simulink model "HybridControllerD3D3_1Act"  (Simulink 8.1)
settings: Solver=FixedStepDiscrete  SolverMode=SingleTasking  StartTime=0.0  StopTime=inf  FixedStep=0.001  MaxStep=.1  RelTol=1e-3
PreLoadFcn:
  | initializeSimulation
PostLoadFcn:
  | , if any(exist('dsrtsu_mdlpostloadfcn', 'file') == [2, 3, 6]), try dsrtsu_mdlpostloadfcn('Execute', bdroot); catch fprintf('Error in PostLoadFcn (dsrtsu_mdlpostloadfcn) for model "%s":\n %s\n', bdroot, lasterr); end, end,
values from neighbouring files (symbols this model uses):
  nAct = 1    [initializeSimulation.m]
  newTarget = 0    [initializeSimulation.m]
  targDsp = zeros(1,nAct)    [initializeSimulation.m]
undefined symbols (not defined in the file): HybridCtrlParameters
libraries: simulink x4, HybridSimLib x3, rtilib1104 x2
CloseFcn:
  | rtwprivate ssgencode ModelCloseRequest HybridController2
settings Model: DSRTSU_INTERNAL_RTI_VER=420  DSRTSU_INTERNAL_RTI_TYPE=rti1104  DSRTSU_INTERNAL_RTIFPGA=10  Creator=Andreas Schellenberg  LastModifiedBy=RTHS Experimentalist  ExtModeAutoUpdateStatusClock=off  TunableVars=newTarget,targDsp  TunableVarsStorageClass=ExportedGlobal,ExportedGlobal  TunableVarsTypeQualifier=volatile,volatile  BufferReuse=off
settings DataIOCC: LimitDataPoints=off  SaveOutput=off  SignalLogging=off  SaveTime=off  SignalLoggingName=sigsOut
settings OptimizationCC: BlockReduction=off  ConditionallyExecuteInputs=off  InlineParams=on  OptimizeBlockIOStorage=off  BufferReuse=off  ExpressionFolding=off  FoldNonRolledExpr=off  LocalBlockOutputs=off  StateBitsets=on  DataBitsets=on  UseTempVars=on  InitFltsAndDblsToZero=on  EfficientFloat2IntCast=on
settings DebuggingCC: SaveWithParameterizedLinksMsg=none  CheckSSInitialOutputMsg=off  SolverPrmCheckMsg=none  StrictBusMsg=None
settings HardwareCC: ProdIntDivRoundTo=Zero  ProdEndianess=BigEndian  ProdHWDeviceType=Generic->Custom  TargetIntDivRoundTo=Zero  TargetEndianess=BigEndian  TargetHWDeviceType=Generic->Custom
settings SFSimCC: SimCustomHeaderCode="#include \"PredictorCorrector.h\""  SimUserSources=PredictorCorrector.c  SimParseCustomCode=off  SimBuildMode=sf_nonincremental_build
settings RTWCC: SystemTargetFile=rti1104.tlc  MakeCommand=make_rti  TemplateMakefile=rti1104.tmf  Description=dSPACE DS1104 Hardware Platform  ProcessScript=rti1104_make_rtw_hook  CustomHeaderCode="#include \"PredictorCorrector.h\""  CustomSource=PredictorCorrector.c  IncludeERTFirstTime=on
settings STFCustomTargetCC: TargetFcnLib=ansi_tfl_tmw.mat  CodeReplacementLibrary=ANSI_C  ParMdlRefBuildCompliant=on  GeneratePreprocessorConditionals=Disable all  LogVarNameModifier=none  SystemTargetFile=rti1104.tlc
settings GRTTargetCC: TargetFcnLib=ansi_tfl_tmw.mat  CompOptLevelCompliant=off  ConcurrentExecutionCompliant=off  LogVarNameModifier=none  MatFileLogging=off  ExtModeMexFile=noextcomm
settings CustomProperty: DataType=RTWOptions_EnumType_C__Program Files_dSPACE RCPHIL 2013-A_MATLAB_RTI_RTI1104_TLC_rti1104_1InitialSimState  Value=STOP
settings EnumStrPairs: String=RUN

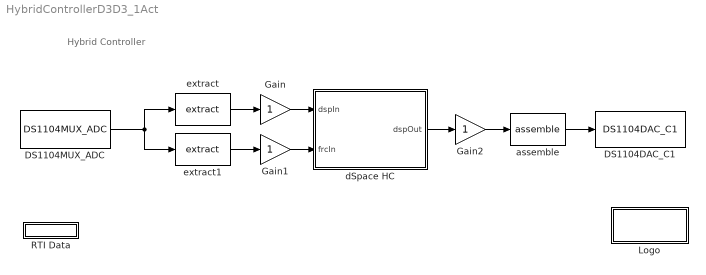
== system HybridControllerD3D3_1Act ==
  note: Hybrid Controller
  DS1104DAC_C1 : rtilib1104/DS1104 MASTER PPC/DS1104DAC_C1  ChannelNo=1  InitValue=0  TermMode=0  TermValue=0  Reserved1=[]  Reserved2=[]  Reserved3=[]  Reserved4=[]  DialogFcn=gui1104dac  UnitName={ 'DS1104DAC_C'}  UnitValues={ 1 }  DSProperties=struct('RTI',struct('Version',uint32(1),'BlockType',struct('isSLSource',uint8(0),'isSLSink',uint8(1),'isHWSource',uint8(0),'isHWSink',uint8(1),'isSetup',uint8(0),'isInline',uint8(1),'isNonInline',uint8(0),'isInterrupt',uint8(0),'isChannelwise',uint8(1)),'IOBoardType','DS1104MASTER','UnitType','DAC','Identifier','DAC','DialogType','ML','BlockSet','NONE','SlaveProcessor','NONE'))
  DS1104MUX_ADC : rtilib1104/DS1104 MASTER PPC/DS1104MUX_ADC  ChannelNos=[1 3]  TriggerMode=0  Reserved1=[]  Reserved2=[]  Reserved3=[]  Reserved4=[]  DialogFcn=gui1104mux_adc  UnitName={ 'DS1104MUX_ADC' }  UnitValues={ [] }  DSProperties=struct('RTI',struct('Version',uint32(1),'BlockType',struct('isSLSource',uint8(1),'isSLSink',uint8(0),'isHWSource',uint8(1),'isHWSink',uint8(0),'isSetup',uint8(0),'isInline',uint8(1),'isNonInline',uint8(0),'isInterrupt',uint8(0),'isChannelwise',uint8(0)),'IOBoardType','DS1104MASTER','UnitType','ADC','Identifier','ADCMUX','DialogType','ML','BlockSet','NONE','SlaveProcessor','NONE'))
  Gain : Gain  SaturateOnIntegerOverflow=on  OutDataTypeStr=Inherit: Same as input  ParamDataTypeStr=Inherit: Same as input
  Gain1 : Gain  SaturateOnIntegerOverflow=on  OutDataTypeStr=Inherit: Same as input  ParamDataTypeStr=Inherit: Same as input
  Gain2 : Gain  SaturateOnIntegerOverflow=on  OutDataTypeStr=Inherit: Same as input  ParamDataTypeStr=Inherit: Same as input
  Logo : Subsystem  mask(dSPACE){EmptyParameter=[]}
      mask prompts: EmptyParameter "Mask Parameter 1:"
      settings: OpenFcn=;
      mask Display: image(imread('rti_mdl_dslogo.tif'));
  RTI Data : Subsystem  Tag=struct('RTIDataServer',struct('RTIDataServerVs','2','RTIModelDescription','struct(''main'',''HybridControllerD3D3_1Act'',''sub'','''',''isMp'',0)'))  LoadFcn="if exist('rtidc'), try,  rtidc('DataHostBlockClbLoad', gcbh); catch, disp(['Warning: ''LoadFcn'' for RTI Data block failed: ' lasterr]); end, end,"  mask(RTI_DATA_HOST){}
      mask help:
      | RTI Data Block.
      | This block is used by RTI to store internal model-dependent data.
      | Please keep this block on the root level of the model. Deleting this block will result in data loss.
      |
      | NEVER DELETE OR COPY THIS BLOCK!
      settings: CopyFcn="if exist('rtidc'), try,  rtidc('DataHostBlockClbCopy', gcbh); catch, disp(['Warning: ''CopyFcn'' for RTI Data block failed: ' lasterr]); end, end,"  DeleteFcn="if exist('rtidc'), try,  rtidc('DataHostBlockClbDelete', gcbh); catch, disp(['Warning: ''DeleteFcn'' for RTI Data block failed: ' lasterr]); end, end,"  ModelCloseFcn="if exist('rtidc'), try,  rtidc('DataHostBlockClbModelClose', gcbh); catch, disp(['Warning: ''ModelCloseFcn'' for RTI Data block failed: ' lasterr]); end, end,"  PreSaveFcn="if exist('rtidc'), try,  rtidc('DataHostBlockClbPreSave', gcbh); catch, disp(['Warning: ''PreSaveFcn'' for RTI Data block failed: ' lasterr]); end, end,"  PostSaveFcn="if exist('rtidc'), try,  rtidc('DataHostBlockClbPostSave', gcbh); catch, disp(['Warning: ''PostSaveFcn'' for RTI Data block failed: ' lasterr]); end, end,"  NameChangeFcn="if exist('rtidc'), try,  rtidc('DataHostBlockClbNameChange', gcbh); catch, disp(['Warning: ''NameChangeFcn'' for RTI Data block failed: ' lasterr]); end, end,"
      mask Help:
      | RTI Data Block.
      | This block is used by RTI to store internal model-dependent data.
      | Please keep this block on the root level of the model. Deleting this block will result in data loss.
      | 
      | NEVER DELETE OR COPY THIS BLOCK!
      mask Display:
      | text(0.5, 0.5, 'RTI Data', 'HorizontalAlignment', 'center');
      | plot([1 0]);
  assemble : HybridSimLib/Signal Routing/assemble  id=1  size=nAct
  dSpace HC : Subsystem  mask(Hybrid Controller: D3/D3){nAct=1, dtInt=HybridCtrlParameters.dtInt, dtSim=HybridCtrlParameters.dtSim, dtCon=HybridCtrlParameters.dtCon, N=HybridCtrlParameters.N, iDelay=HybridCtrlParameters.iDelay, dspLim=HybridCtrlParameters.dspLim, velLim=HybridCtrlParameters.velLim}
      mask prompts: nAct "Number of Actuators: nAct"; dtInt "Integration time step: dtInt"; dtSim "Simulation time step: dtSim"; dtCon "Controller time step: dtCon"; N "Maximum number of substeps: N"; iDelay "Number of delay steps: iDelay"; dspLim "Displacement limit: dspLim"; velLim "Velocity limit: velLim"
      mask help: Hybrid Controller using C0-continuous cubic Lagrange interpolation for prediction and correction
      mask Display: disp('dSpace\nHybrid Controller\n(D3/D3)')
  extract : HybridSimLib/Signal Routing/extract  id=1  size=2*nAct
  extract1 : HybridSimLib/Signal Routing/extract  id=2  size=2*nAct
  wires:
  dSpace HC/1(dspOut) -> Gain2/1
  Gain/1 -> dSpace HC/1(dspIn)
  Gain1/1 -> dSpace HC/2(frcIn)
  DS1104MUX_ADC/1 -> extract/1, extract1/1
  Gain2/1 -> assemble/1
  extract/1 -> Gain/1
  extract1/1 -> Gain1/1
  assemble/1 -> DS1104DAC_C1/1

== system HybridControllerD3D3_1Act/Logo ==
  note: $Workfile: demo1104_analog.mdl $
  note: $Date: 2011-05-22 14:17:07 -0700 (Sun, 22 May 2011) $
  note: $Revision: 314 $

== system HybridControllerD3D3_1Act/RTI Data ==
  RTI Data Store : Subsystem  Tag="struct('private',struct('version',struct('dsVer',uint32(2),'dsVerCreation',uint32(2),'RTI',struct('ver','4.1a3','type','RTI1104')),'access',struct('type','Model','isPerm',1,'created',['13-Feb-2001 14:58:17'],'modified',['01-Oct-2013 23:15:47'],'location','')),'public',struct('main',struct('data',[]),'sub',struct('name',{{'HybridControllerD3D3_1Act'}},'data',{{struct('TH',struct('thTaskInfo',struct('taskType',{'TIMER','HWINT','TMRINT','SWINT','GLINT'},'tasksNumOf',{1,0,0,0,0},'srcIds',{{'TIMERA'},{},{},{},{}},'taskNames',{{['Timer Task 1']},{},{},{},{}})),'th_tc',struct('dataType','TASK','taskGroupId','','taskGroupList',{{}},'taskSchedulingPolicy','FCFS','taskType','TIMER','blkh',-1,'srcId','TIMERA','srcSgnName',['Timer A interrupt'],'srcCpuName','','taskName',['Timer Task 1  [0.001] s'],'taskNameDisplayExt','','smplTime',0.001,'smplTimeOffs',0,'hasFixedPriority',0,'priority',1,'hasFixedOvc',0,'ovcType',1,'ovcMax',0),'tc_th',struct('dataType','TASK','taskGroupId','','taskGroupList',{{}},'taskSchedulingPolicy','FCFS','taskType','TIMER','blkh',-1,'srcId','TIMERA','srcSgnName',['Timer A interrupt'],'srcCpuName','','taskName',['Timer Task 1  [0.001] s'],'taskNameDisplayExt','','smplTime',0.001,'smplTimeOffs',0,'hasFixedPriority',0,'priority',1,'hasFixedOvc',0,'ovcType',1,'ovcMax',0))}})))"  mask(RTI_DATA_STORE){}
      mask help:
      | RTI Data Store Block. This block is used by RTI to store internal model dependent data. Deleting this block will result in data loss.
      |
      | NEVER DELETE, COPY, OR MODIFY THIS BLOCK!
      mask Help:
      | RTI Data Store Block. This block is used by RTI to store internal model dependent data. Deleting this block will result in data loss.
      | 
      | NEVER DELETE, COPY, OR MODIFY THIS BLOCK!
      mask Display: text(0.5, 0.5, ' ', 'HorizontalAlignment', 'center');

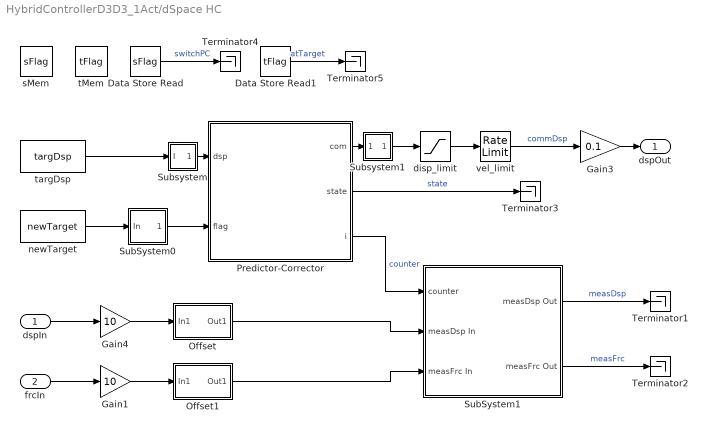
== system HybridControllerD3D3_1Act/dSpace HC ==
  dspIn : Inport
  frcIn : Inport  Port=2
  Data Store Read : DataStoreRead  DataStoreName=sFlag  SampleTime=dtCon
  Data Store Read1 : DataStoreRead  DataStoreName=tFlag  SampleTime=dtCon
  Gain1 : Gain  Gain=10  SaturateOnIntegerOverflow=on  OutDataTypeStr=Inherit: Same as input  ParamDataTypeStr=Inherit: Same as input
  Gain3 : Gain  Gain=0.1  SaturateOnIntegerOverflow=on  OutDataTypeStr=Inherit: Same as input  ParamDataTypeStr=Inherit: Same as input
  Gain4 : Gain  Gain=10  SaturateOnIntegerOverflow=on  OutDataTypeStr=Inherit: Same as input  ParamDataTypeStr=Inherit: Same as input
  Offset : Subsystem  mask(Signal Offset){nS=nAct, nOffset=1024, dt=dtCon}
      mask prompts: nS "Number of Signals: nS"; nOffset "Number of samples to initialize offset: nOffset"; dt "Sample time: dt"
      mask help: Offset signal by average of signal over initial number of samples
      mask Display: fprintf('Signal\nOffset')
  Offset1 : Subsystem  mask(Signal Offset){nS=nAct, nOffset=1024, dt=dtCon}
      mask prompts: nS "Number of Signals: nS"; nOffset "Number of samples to initialize offset: nOffset"; dt "Sample time: dt"
      mask help: Offset signal by average of signal over initial number of samples
      mask Display: fprintf('Signal\nOffset')
  Predictor-Corrector : Stateflow chart  TreatAsAtomicUnit=on
  SubSystem0 : Subsystem
  SubSystem1 : Subsystem
  Subsystem : Subsystem
      mask Display: disp('I/O')
  Subsystem1 : Subsystem
      mask Display: disp('I/O')
  Terminator{1..5} (5 alike) : Terminator
  disp_limit : Saturate  UpperLimit=dspLim  LowerLimit=-dspLim
  newTarget : Constant  Value=newTarget  OutDataTypeStr=uint32  SampleTime=dtCon
  sMem : DataStoreMemory  DataStoreName=sFlag  OutDataTypeStr=uint32
  tMem : DataStoreMemory  DataStoreName=tFlag  OutDataTypeStr=uint32
  targDsp : Constant  Value=targDsp  SampleTime=dtCon
  vel_limit : RateLimiter  RisingSlewLimit=velLim  FallingSlewLimit=-velLim
  dspOut : Outport
  wires:
  frcIn/1 -> Gain1/1
  dspIn/1 -> Gain4/1
  SubSystem1/2(measFrc Out) -> Terminator2/1  "measFrc"
  SubSystem1/1(measDsp Out) -> Terminator1/1  "measDsp"
  Predictor-Corrector/3(i) -> SubSystem1/1(counter)  "counter"
  Predictor-Corrector/2(state) -> Terminator3/1  "state"
  Offset/1(Out1) -> SubSystem1/2(measDsp In)
  newTarget/1 -> SubSystem0/1(In)
  targDsp/1 -> Subsystem/1(I)
  Offset1/1(Out1) -> SubSystem1/3(measFrc In)
  disp_limit/1 -> vel_limit/1
  vel_limit/1 -> Gain3/1  "commDsp"
  Predictor-Corrector/1(com) -> Subsystem1/1(In)
  Gain3/1 -> dspOut/1
  Gain4/1 -> Offset/1(In1)
  Gain1/1 -> Offset1/1(In1)
  Data Store Read/1 -> Terminator4/1  "switchPC"
  Data Store Read1/1 -> Terminator5/1  "atTarget"
  Subsystem1/1(Out) -> disp_limit/1
  SubSystem0/1(Out) -> Predictor-Corrector/2(flag)
  Subsystem/1(O) -> Predictor-Corrector/1(dsp)

== system HybridControllerD3D3_1Act/RTI Data/RTI Data Store ==
  RTI Data Store : Subsystem  mask(RTI_DATA_STORE){}
      mask help:
      | RTI Data Store Block. This block is used by RTI to store internal model dependent data. Deleting this block will result in data loss.
      |
      | NEVER DELETE, COPY, OR MODIFY THIS BLOCK!
      mask Help:
      | RTI Data Store Block. This block is used by RTI to store internal model dependent data. Deleting this block will result in data loss.
      | 
      | NEVER DELETE, COPY, OR MODIFY THIS BLOCK!
      mask Display: text(0.5, 0.5, ' ', 'HorizontalAlignment', 'center');

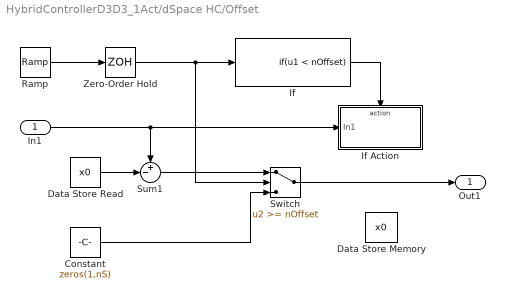
== system HybridControllerD3D3_1Act/dSpace HC/Offset ==
  In1 : Inport
  Constant : Constant  Value=zeros(1,nS)
  Data Store Memory : DataStoreMemory  DataStoreName=x0  InitialValue=zeros(1,nS)  OutDataTypeStr=double
  Data Store Read : DataStoreRead  DataStoreName=x0  SampleTime=dt
  If : If  IfExpression=u1 < nOffset  ShowElse=off
  If Action : Subsystem  TreatAsAtomicUnit=on
  Ramp : simulink/Sources/Ramp  slope=1/dt  start=0  X0=0
  Sum1 : Sum  Inputs=+-|  SaturateOnIntegerOverflow=on  InputSameDT=on  OutDataTypeStr=Inherit: Same as first input
  Switch : Switch  Threshold=nOffset  SaturateOnIntegerOverflow=on  InputSameDT=on
  Zero-Order Hold : ZeroOrderHold  SampleTime=dt
  Out1 : Outport
  wires:
  Switch/1 -> Out1/1
  Sum1/1 -> Switch/1
  Data Store Read/1 -> Sum1/2
  In1/1 -> If Action/1(In1), Sum1/1
  Constant/1 -> Switch/3
  Zero-Order Hold/1 -> Switch/2, If/1
  If/1 -> If Action/Action
  Ramp/1 -> Zero-Order Hold/1

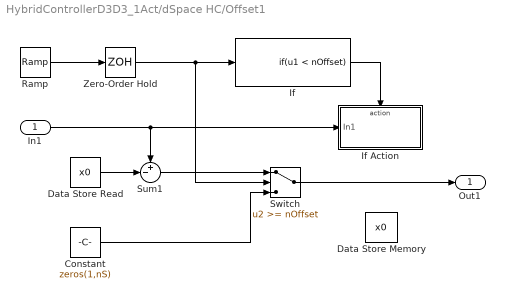
== system HybridControllerD3D3_1Act/dSpace HC/Offset1 ==
  In1 : Inport
  Constant : Constant  Value=zeros(1,nS)
  Data Store Memory : DataStoreMemory  DataStoreName=x0  InitialValue=zeros(1,nS)  OutDataTypeStr=double
  Data Store Read : DataStoreRead  DataStoreName=x0  SampleTime=dt
  If : If  IfExpression=u1 < nOffset  ShowElse=off
  If Action : Subsystem  TreatAsAtomicUnit=on
  Ramp : simulink/Sources/Ramp  slope=1/dt  start=0  X0=0
  Sum1 : Sum  Inputs=+-|  SaturateOnIntegerOverflow=on  InputSameDT=on  OutDataTypeStr=Inherit: Same as first input
  Switch : Switch  Threshold=nOffset  SaturateOnIntegerOverflow=on  InputSameDT=on
  Zero-Order Hold : ZeroOrderHold  SampleTime=dt
  Out1 : Outport
  wires:
  Switch/1 -> Out1/1
  Sum1/1 -> Switch/1
  Data Store Read/1 -> Sum1/2
  In1/1 -> If Action/1(In1), Sum1/1
  Constant/1 -> Switch/3
  Zero-Order Hold/1 -> Switch/2, If/1
  If/1 -> If Action/Action
  Ramp/1 -> Zero-Order Hold/1

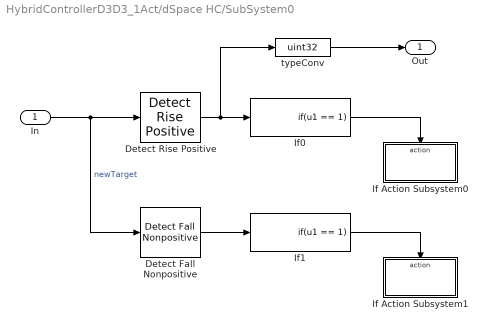
== system HybridControllerD3D3_1Act/dSpace HC/SubSystem0 ==
  In : Inport
  Detect Fall Nonpositive : simulink/Logic and Bit Operations/Detect Fall Nonpositive  vinit=0  InputProcessing=Inherited  OutDataTypeStr=uint8
  Detect Rise Positive : simulink/Logic and Bit Operations/Detect Rise Positive  vinit=0  InputProcessing=Inherited  OutDataTypeStr=uint8
  If Action Subsystem0 : Subsystem  TreatAsAtomicUnit=on
  If Action Subsystem1 : Subsystem  TreatAsAtomicUnit=on
  If0 : If  IfExpression=u1 == 1  ShowElse=off
  If1 : If  IfExpression=u1 == 1  ShowElse=off
  typeConv : DataTypeConversion  OutDataTypeStr=uint32  SaturateOnIntegerOverflow=on  RndMeth=Zero
  Out : Outport
  wires:
  In/1 -> Detect Rise Positive/1, Detect Fall Nonpositive/1  "newTarget"
  Detect Rise Positive/1 -> If0/1, typeConv/1
  Detect Fall Nonpositive/1 -> If1/1
  If1/1 -> If Action Subsystem1/Action
  If0/1 -> If Action Subsystem0/Action
  typeConv/1 -> Out/1

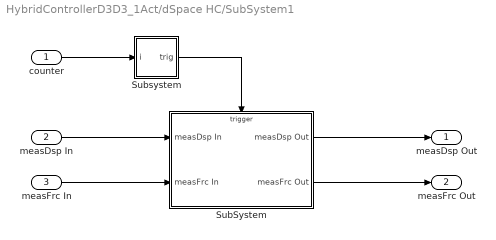
== system HybridControllerD3D3_1Act/dSpace HC/SubSystem1 ==
  counter : Inport
  measDsp In : Inport  Port=2
  measFrc In : Inport  Port=3
  SubSystem : Subsystem  TreatAsAtomicUnit=on
  Subsystem : Subsystem
  measDsp Out : Outport
  measFrc Out : Outport  Port=2
  wires:
  SubSystem/2(measFrc Out) -> measFrc Out/1
  measFrc In/1 -> SubSystem/2(measFrc In)
  SubSystem/1(measDsp Out) -> measDsp Out/1
  measDsp In/1 -> SubSystem/1(measDsp In)
  counter/1 -> Subsystem/1(i)
  Subsystem/1(trig) -> SubSystem/Trigger

== system HybridControllerD3D3_1Act/dSpace HC/Subsystem ==
  I : Inport  PortDimensions=nAct
  Dummy Aug : Mux  Inputs=[nAct 1]
  Dummy Zero : Constant  Value=0  OutDataTypeStr=double  SampleTime=dtCon
  O : Outport  PortDimensions=nAct+1
  wires:
  Dummy Zero/1 -> Dummy Aug/2
  I/1 -> Dummy Aug/1
  Dummy Aug/1 -> O/1

== system HybridControllerD3D3_1Act/dSpace HC/Subsystem1 ==
  In : Inport  PortDimensions=nAct+1
  Dummy Trn : Demux  Outputs=[nAct 1]
  Terminator3 : Terminator
  Out : Outport  PortDimensions=nAct
  wires:
  Dummy Trn/2 -> Terminator3/1
  Dummy Trn/1 -> Out/1
  In/1 -> Dummy Trn/1

== system HybridControllerD3D3_1Act/RTI Data/RTI Data Store/RTI Data Store ==
  RTI Data Store : Subsystem  mask(RTI_DATA_STORE){}
      mask help:
      | RTI Data Store Block. This block is used by RTI to store internal model dependent data. Deleting this block will result in data loss.
      |
      | NEVER DELETE, COPY, OR MODIFY THIS BLOCK!
      mask Help:
      | RTI Data Store Block. This block is used by RTI to store internal model dependent data. Deleting this block will result in data loss.
      | 
      | NEVER DELETE, COPY, OR MODIFY THIS BLOCK!
      mask Display: text(0.5, 0.5, ' ', 'HorizontalAlignment', 'center');

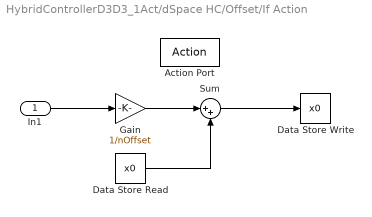
== system HybridControllerD3D3_1Act/dSpace HC/Offset/If Action ==
  In1 : Inport
  Action Port : ActionPort  PropagateVarSize=During execution  ActionType=then
  Data Store Read : DataStoreRead  DataStoreName=x0  SampleTime=dt
  Data Store Write : DataStoreWrite  DataStoreName=x0
  Gain : Gain  Gain=1/nOffset  SaturateOnIntegerOverflow=on  OutDataTypeStr=Inherit: Same as input  ParamDataTypeStr=Inherit: Same as input
  Sum : Sum  Inputs=|++  SaturateOnIntegerOverflow=on  InputSameDT=on  OutDataTypeStr=Inherit: Same as first input
  wires:
  Data Store Read/1 -> Sum/2
  Sum/1 -> Data Store Write/1
  Gain/1 -> Sum/1
  In1/1 -> Gain/1

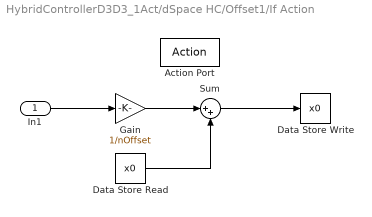
== system HybridControllerD3D3_1Act/dSpace HC/Offset1/If Action ==
  In1 : Inport
  Action Port : ActionPort  PropagateVarSize=During execution  ActionType=then
  Data Store Read : DataStoreRead  DataStoreName=x0  SampleTime=dt
  Data Store Write : DataStoreWrite  DataStoreName=x0
  Gain : Gain  Gain=1/nOffset  SaturateOnIntegerOverflow=on  OutDataTypeStr=Inherit: Same as input  ParamDataTypeStr=Inherit: Same as input
  Sum : Sum  Inputs=|++  SaturateOnIntegerOverflow=on  InputSameDT=on  OutDataTypeStr=Inherit: Same as first input
  wires:
  Data Store Read/1 -> Sum/2
  Sum/1 -> Data Store Write/1
  Gain/1 -> Sum/1
  In1/1 -> Gain/1

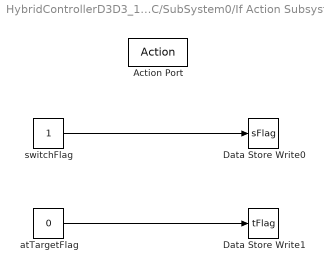
== system HybridControllerD3D3_1Act/dSpace HC/SubSystem0/If Action Subsystem0 ==
  Action Port : ActionPort  PropagateVarSize=During execution  ActionType=then
  Data Store Write0 : DataStoreWrite  DataStoreName=sFlag
  Data Store Write1 : DataStoreWrite  DataStoreName=tFlag
  atTargetFlag : Constant  Value=0  OutDataTypeStr=uint32  SampleTime=dtCon
  switchFlag : Constant  OutDataTypeStr=uint32  SampleTime=dtCon
  wires:
  atTargetFlag/1 -> Data Store Write1/1
  switchFlag/1 -> Data Store Write0/1

== system HybridControllerD3D3_1Act/dSpace HC/SubSystem0/If Action Subsystem1 ==
  Action Port : ActionPort  PropagateVarSize=During execution  ActionType=then
  Data Store Write0 : DataStoreWrite  DataStoreName=sFlag
  switchFlag : Constant  Value=0  OutDataTypeStr=uint32  SampleTime=dtCon
  wires:
  switchFlag/1 -> Data Store Write0/1

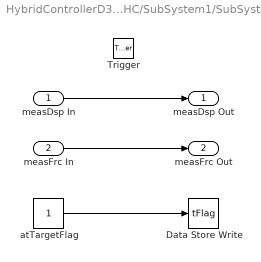
== system HybridControllerD3D3_1Act/dSpace HC/SubSystem1/SubSystem ==
  measDsp In : Inport
  measFrc In : Inport  Port=2
  Trigger : TriggerPort
  Data Store Write : DataStoreWrite  DataStoreName=tFlag
  atTargetFlag : Constant  OutDataTypeStr=uint32  SampleTime=-1
  measDsp Out : Outport  InitialOutput=[0]
  measFrc Out : Outport  Port=2  InitialOutput=[0]
  wires:
  atTargetFlag/1 -> Data Store Write/1
  measFrc In/1 -> measFrc Out/1
  measDsp In/1 -> measDsp Out/1

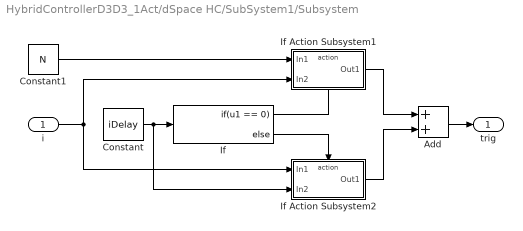
== system HybridControllerD3D3_1Act/dSpace HC/SubSystem1/Subsystem ==
  i : Inport
  Add : Sum
  Constant : Constant  Value=iDelay
  Constant1 : Constant  Value=N
  If : If  IfExpression=u1 == 0
  If Action Subsystem1 : Subsystem  TreatAsAtomicUnit=on
  If Action Subsystem2 : Subsystem  TreatAsAtomicUnit=on
  trig : Outport
  wires:
  Constant/1 -> If/1, If Action Subsystem2/2(In2)
  If/1 -> If Action Subsystem1/Action
  If/2 -> If Action Subsystem2/Action
  If Action Subsystem1/1(Out1) -> Add/1
  If Action Subsystem2/1(Out1) -> Add/2
  Add/1 -> trig/1
  i/1 -> If Action Subsystem1/2(In2), If Action Subsystem2/1(In1)
  Constant1/1 -> If Action Subsystem1/1(In1)

== system HybridControllerD3D3_1Act/RTI Data/RTI Data Store/RTI Data Store/RTI Data Store ==
  RTI Data Store : Subsystem  mask(RTI_DATA_STORE){}
      mask help:
      | RTI Data Store Block. This block is used by RTI to store internal model dependent data. Deleting this block will result in data loss.
      |
      | NEVER DELETE, COPY, OR MODIFY THIS BLOCK!
      mask Help:
      | RTI Data Store Block. This block is used by RTI to store internal model dependent data. Deleting this block will result in data loss.
      | 
      | NEVER DELETE, COPY, OR MODIFY THIS BLOCK!
      mask Display: text(0.5, 0.5, ' ', 'HorizontalAlignment', 'center');

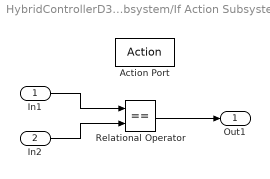
== system HybridControllerD3D3_1Act/dSpace HC/SubSystem1/Subsystem/If Action Subsystem1 ==
  In1 : Inport
  In2 : Inport  Port=2
  Action Port : ActionPort  ActionType=then
  Relational Operator : RelationalOperator  Operator===  OutDataTypeStr=boolean
  Out1 : Outport
  wires:
  Relational Operator/1 -> Out1/1
  In1/1 -> Relational Operator/1
  In2/1 -> Relational Operator/2

== system HybridControllerD3D3_1Act/dSpace HC/SubSystem1/Subsystem/If Action Subsystem2 ==
  In1 : Inport
  In2 : Inport  Port=2
  Action Port : ActionPort  ActionType=else
  Relational Operator : RelationalOperator  Operator===  OutDataTypeStr=boolean
  Out1 : Outport
  wires:
  Relational Operator/1 -> Out1/1
  In1/1 -> Relational Operator/1
  In2/1 -> Relational Operator/2

== system HybridControllerD3D3_1Act/RTI Data/RTI Data Store/RTI Data Store/RTI Data Store/RTI Data Store ==

== stateflow chart dSpace HC/Predictor-Corrector ==
  state HybridController [parallel]
    settings: executionOrder=1
    state Predict
      en: state = 1;
      en: diSD = 1;
      en: i = 1; iSD = 0;
      en: predictP3(com,i/N);
      du: i++;
      du: predictP3(com,i/N);
    state Initialize
      en: i = 0; iSD = 0;
      en: diSD = 1;
      en: initData(nAct,dtCon);
      en: zeroDsp(com);
    state AutoSlowDown
      en: state = 2;
      en: diSD = 4-i/(0.2*N);
      en: i += diSD; iSD = i;
      en: predictP3(com,i/N);
      du: diSD = 4-i/(0.2*N);
      du: i += diSD; iSD = i;
      du: predictP3(com,i/N);
    state Correct
      en: state = 0;
      en: setCurDsp(com,i/N);
      en: dspLocal = dsp; setNewDsp(dspLocal);
      en: di = min(max(diSD+1/(0.2*N)*(i-iSD),0.001),1);
      en: i = min(i+di,N);
      en: correctP3(com,i/N);
      du: di = min(max(diSD+1/(0.2*N)*(i-iSD),0.001),1);
      du: i = min(i+di,N);
      du: correctP3(com,i/N);
    Correct -> Predict [order 1] : [i>=N && flag!=1]
    (default) -> Initialize
    Initialize -> Correct : [flag==1]
    Correct -> Correct [order 2] : [flag==1]
        | {i=0; iSD=0; diSD=1}
    AutoSlowDown -> Correct : [flag==1]
    Predict -> Correct [order 2] : [flag==1]
    Predict -> AutoSlowDown [order 1] : [i>=0.6*N && flag!=1]
  data: dsp input double size=nAct+1; flag input uint32; com output double size=nAct+1; state output uint32; i output double; N local double; nAct parameter uint32 =1; di local double; diSD local double; iSD local double; dspLocal local double size=nAct+1
